simulink subsystem "currentControlWithFF"  (R2023b)
settings: Solver=VariableStepAuto  StartTime=0.0  StopTime=10.0  RelTol=1e-3
undefined symbols (not defined in the file): ctrl_tsk_st, hpfratio
libraries: spsFirstOrderFilterLib x1
settings Model: DataDictionary=fmuGenerationDictionay.sldd  EnableAccessToBaseWorkspace=off  Creator=Veimar  LastModifiedBy=Veimar

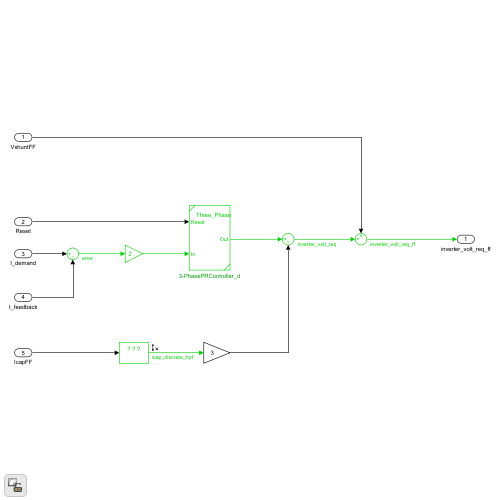
[thumbnail: Simulink's stored preview of the top-level diagram]
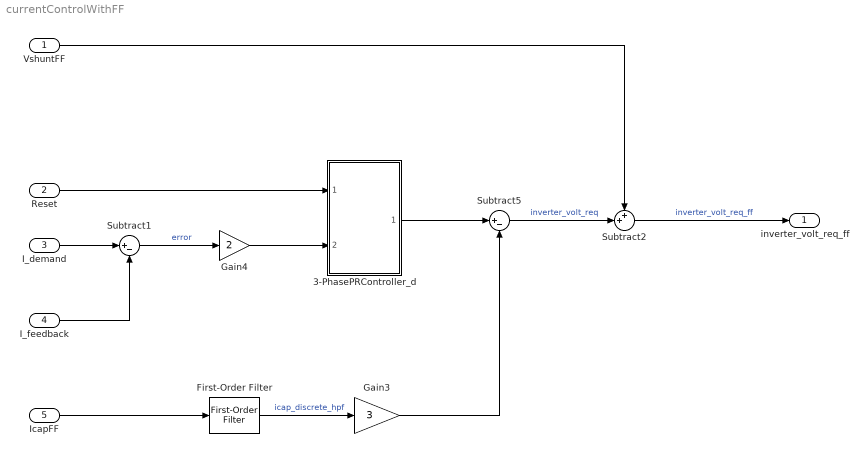
== system currentControlWithFF ==
  VshuntFF : Inport  OutDataTypeStr=single  PortDimensions=3
  Reset : Inport  Port=2  OutDataTypeStr=boolean  PortDimensions=3
  I_demand : Inport  Port=3  OutDataTypeStr=single  PortDimensions=3
  I_feedback : Inport  Port=4  OutDataTypeStr=single  PortDimensions=3
  IcapFF : Inport  Port=5  OutDataTypeStr=single  PortDimensions=3
  3-PhasePRController_d : Subsystem  ReferencedSubsystem=Three_PhasePRController
  First-Order Filter : spsFirstOrderFilterLib/First-Order Filter  FilterType=Highpass  Tc=ctrl_tsk_st/hpfratio  Ts=ctrl_tsk_st  Initialize=off  Vac_Init=[0, 0, 60]  Vdc_Init=0  PlotResponse=off  FreqRange="[0,  200,  1]"
  Gain3 : Gain  Gain=3
  Gain4 : Gain  Gain=2
  Subtract1 : Sum  Inputs=|+-
  Subtract2 : Sum  Inputs=++|
  Subtract5 : Sum  Inputs=|+-
  inverter_volt_req_ff : Outport  OutDataTypeStr=single  PortDimensions=3
  wires:
  Subtract5/1 -> Subtract2/2  "inverter_volt_req"
  First-Order Filter/1 -> Gain3/1  "icap_discrete_hpf"
  Gain4/1 -> 3-PhasePRController_d/2
  Subtract1/1 -> Gain4/1  "error"
  3-PhasePRController_d/1 -> Subtract5/1
  VshuntFF/1 -> Subtract2/1
  Gain3/1 -> Subtract5/2
  I_demand/1 -> Subtract1/1
  IcapFF/1 -> First-Order Filter/1
  I_feedback/1 -> Subtract1/2
  Reset/1 -> 3-PhasePRController_d/1
  Subtract2/1 -> inverter_volt_req_ff/1  "inverter_volt_req_ff"
